simulink model "simulation"  (R2022a)
settings: Solver=VariableStepAuto  StartTime=0.0  StopTime=inf  RelTol=1e-3
settings Model: Creator=jeeva  LastModifiedBy=shobh

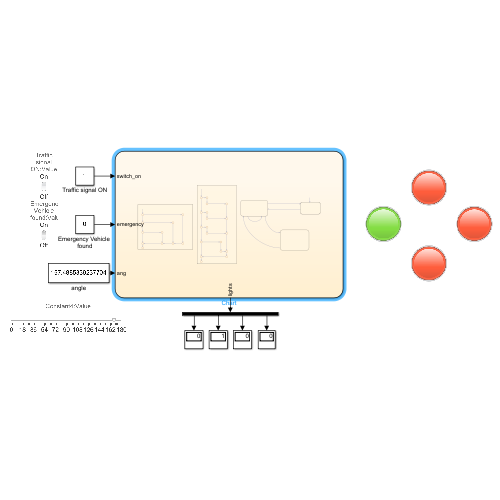
[thumbnail: Simulink's stored preview of the top-level diagram]
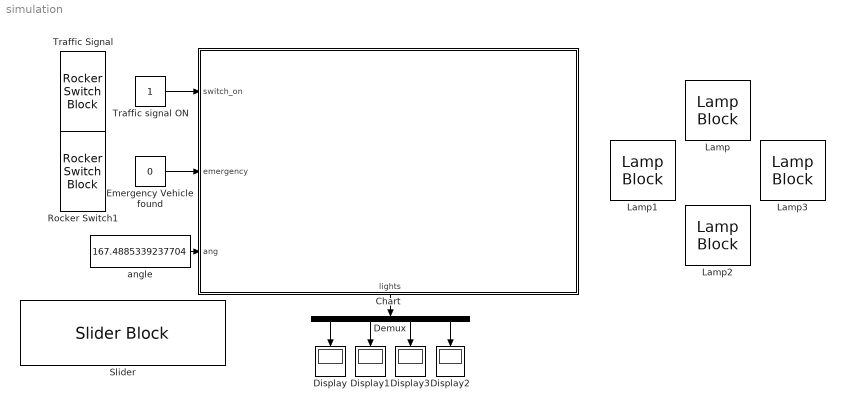
== system simulation ==
  Chart : Stateflow chart  TreatAsAtomicUnit=on
      settings: PortSchema="{\"entries\":[{\"content\":{\"sides\":[{\"content\":{\"connectorIds\":[\"In1\",\"In2\",\"In3\"]},\"type\":\"ConnectorPlacement.EquallySpacedRectSide\",\"uuid\":\"ef1ac283-7c40-4782-9fdd-a35b7e513957\"},{\"content\":{\"connectorIds\":[],\"side\":\"RIGHT\"},\"type\":\"ConnectorPlacement.EquallySpacedRectSide\",\"uuid\":\"3a547a36-f081-4294-9730-36eea3362598\"},{\"content\":{\"connectorIds\":[],\"side\":\"TOP\"},\"type\":\"ConnectorPlacement.EquallySpacedRectSide\",\"uuid\":\"7b6ff503-3baa-490e-a01c-ee1c44c67fcf\"},{\"content\":{\"connectorIds\":[\"Out1\"],\"side\":\"BOTTOM\"},\"type\":\"ConnectorPlacement.EquallySpacedRectSide\",\"uuid\":\"c371e26e-7278-4635-ba47-5b12d85dd724\"}]},\"type\":\"ConnectorPlacement.EquallySpacedConnector\",\"uuid\":\"07f18f62-5d2b-42f1-8d6c-740611540770\"}],\"packageUris\":[\"http://schema.mathworks.com/mf0/Connector/R2020b\"],\"version\":\"1.0\"}"
  Demux : Demux
  Display{,1..3} (4 alike) : Display
  Emergency Vehicle found : Constant  Value=0
  Lamp{,1..3} (4 alike) : LampBlock  LabelPosition=Hide
  Rocker Switch1 : RockerSwitchBlock
      settings: Values={{'Off', 'On'}, [0 1]}
  Slider : SliderBlock  ScaleMax=180
  Traffic Signal : RockerSwitchBlock
      settings: Values={{'Off', 'On'}, [0 1]}
  Traffic signal ON : Constant
  angle : Constant  Value=167.4885339237704
  wires:
  Traffic signal ON/1 -> Chart/1(switch_on)
  angle/1 -> Chart/3(ang)
  Demux/1 -> Display/1
  Demux/2 -> Display1/1
  Demux/3 -> Display3/1
  Demux/4 -> Display2/1
  Emergency Vehicle found/1 -> Chart/2(emergency)
  Chart/1(lights) -> Demux/1

== stateflow chart simulation/Chart ==
  state lights = changeLights(counter4) [function]
    (default) -> (junction 83)
    (junction 83) -> (junction 84) [order 1] : [counter4 == 0]
    (junction 83) -> (junction 87) [order 2]
    (junction 84) -> (junction 85) : {lights = [1 0 0 0];}
    (junction 85) -> (junction 86)
    (junction 86) -> (junction 90)
    (junction 87) -> (junction 88) [order 1] : [counter4 == 1]
    (junction 87) -> (junction 91) [order 2]
    (junction 88) -> (junction 89) : {lights = [0 1 0 0];}
    (junction 89) -> (junction 90)
    (junction 90) -> (junction 94)
    (junction 91) -> (junction 92) [order 1] : [counter4 == 2]
    (junction 91) -> (junction 95) [order 2]
    (junction 92) -> (junction 93) : {lights = [0 0 1 0];}
    (junction 93) -> (junction 94)
    (junction 94) -> (junction 98)
    (junction 95) -> (junction 96) [order 1] : [counter4 == 3]
    (junction 95) -> (junction 99) [order 2] : {lights = [0 0 0 0];}
    (junction 96) -> (junction 97) : {lights = [0 0 0 1];}
    (junction 97) -> (junction 98)
    (junction 98) -> (junction 100)
    (junction 100) -> (junction 99)
    (junction 99) -> (junction 101)
  state On
    entry:
    counter = mod(counter + 1,20)
    counter4 = floor(counter/5);
    lights = changeLights(counter4);
    pause(1);
  state Off
    lights = [2,2,2,2];
  state pos = positionTrack(angle) [function]
    (default) -> (junction 39)
    (junction 39) -> (junction 40) [order 1] : [angle < 60]
    (junction 39) -> (junction 41) [order 2]
    (junction 40) -> (junction 48) : {pos = 0;}
    (junction 41) -> (junction 42) [order 1] : [angle < 120 && angle > 60]
    (junction 41) -> (junction 43) [order 2]
    (junction 42) -> (junction 47) : {pos = 1;}
    (junction 43) -> (junction 44) [order 1] : [angle > 180]
    (junction 43) -> (junction 45) [order 2] : {pos = 3;}
    (junction 44) -> (junction 46) : {pos = 2;}
    (junction 46) -> (junction 45)
    (junction 47) -> (junction 46)
    (junction 48) -> (junction 47)
    (junction 45) -> (junction 49)
  state EmergencyFound
    entry: lights = [0, 1, 0, 0];
  (default) -> Off
  On -> Off [order 1] : [switch_on == 0]
  Off -> On : [switch_on == 1]{counter = 0}
  EmergencyFound -> On : [positionTrack(ang) == 2]
  On -> On [order 2] : [~emergency]
  On -> EmergencyFound [order 3] : [emergency]
  data: counter4 function_input; lights function_output; angle function_input; pos function_output; lights output; switch_on input; counter local; emergency input; ang input; counter4 local
